simulink model "gm_sampleModel1787_sub"  (R2023a)
settings: Solver=VariableStepAuto  StartTime=0.0  StopTime=10.0  RelTol=1e-3
libraries: simulink x3, hdlsllib x1
settings Model: Creator=user1  LastModifiedBy=user1
settings OptimizationCC: BlockReduction=off  ConditionallyExecuteInputs=off
settings DebuggingCC: InheritedTsInSrcMsg=none

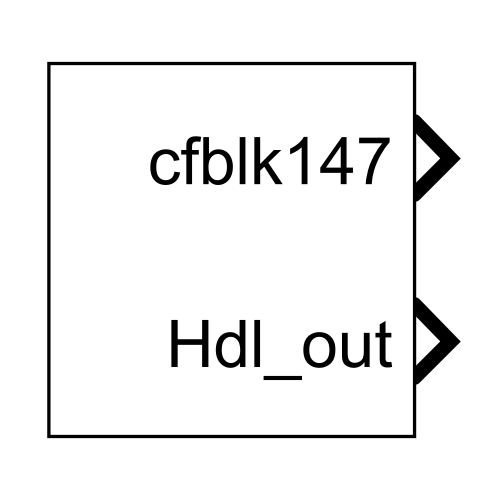
[thumbnail: Simulink's stored preview of the top-level diagram]
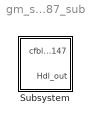
== system gm_sampleModel1787_sub ==
  Subsystem : Subsystem

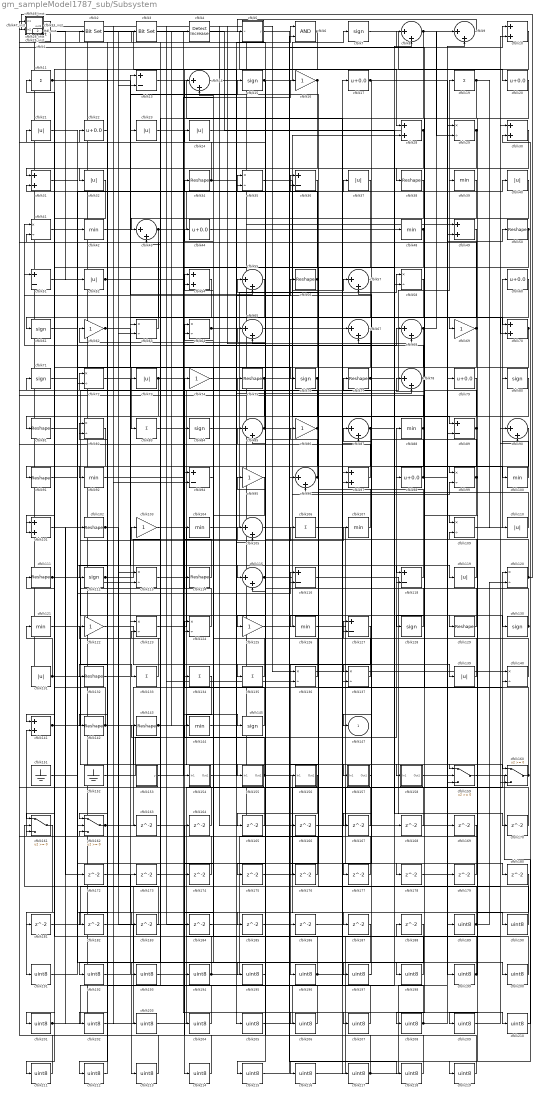
== system gm_sampleModel1787_sub/Subsystem ==
  cfblk1 : hdlsllib/Logic and Bit Operations/Bit Shift  mode=Shift Left Logical  N=0
  cfblk{10,28,30..31,49,54,70,97,101,141} (10 alike) : Sum  OutDataTypeStr=uint8
  cfblk{39,42,48,88,92,100,104,107,121,126,144} (11 alike) : MinMax  OutDataTypeStr=uint8
  cfblk{34,38,50,56,75,77,81,91,102,111,114,129,132,142..143} (15 alike) : Reshape
  cfblk{16,62,69,74,86,95,103,122,125} (9 alike) : Gain  OutDataTypeStr=uint8
  cfblk{8..9,14,43,55,57,65,67..68,78,85,87,90,96,105,115} (16 alike) : Sum  Inputs=|++  OutDataTypeStr=uint8
  cfblk{11,19,83,106,133..135} (7 alike) : Sum  Inputs=+  OutDataTypeStr=uint8
  cfblk108_inst : Subsystem
  cfblk{29,35,41,58,63..64,72,82,99,109,113,120,123..124,136..137,140} (17 alike) : Product  Inputs=*/  OutDataTypeStr=uint8  RndMeth=Zero  SaturateOnIntegerOverflow=on
  cfblk{21,23..24,32,37,40,52,73,110,119,131,139} (12 alike) : Abs  OutDataTypeStr=uint8  SaturateOnIntegerOverflow=off
  cfblk{7,15,61,71,76,80,84,112,128,130,145} (11 alike) : Signum
  cfblk{13,36,51,89,94,116,118,127} (8 alike) : Sum  Inputs=+-  OutDataTypeStr=uint8
  cfblk151 : Ground
  cfblk152 : Ground
  cfblk153 : Subsystem  mask(Counter Free-Running){NumBits=double(16), tsamp=double(-1)}
      mask prompts: NumBits "Simulink:masks:NumberOfBits_MP"; tsamp "Simulink:masks:SampleTime_MP"
      mask help: Simulink:masks:CounterFreeRunning_MD
  cfblk154 : Subsystem
  cfblk155 : Subsystem
  cfblk156 : Subsystem
  cfblk157 : Subsystem
  cfblk158 : Subsystem
  cfblk{159..162} (4 alike) : Switch  OutDataTypeStr=uint8  SaturateOnIntegerOverflow=off  InputSameDT=off
  cfblk{163..170,172..188} (25 alike) : Delay  SampleTime=1
  cfblk{17,20,22,44,60,79,98} (7 alike) : Bias  Bias=0.0  SaturateOnIntegerOverflow=off
  cfblk{189..219} (31 alike) : DataTypeConversion  OutDataTypeStr=uint8  SaturateOnIntegerOverflow=off  RndMeth=Floor
  cfblk18_inst : Subsystem
  cfblk2 : simulink/Logic and Bit Operations/Bit Set  iBit=0
      settings: LibrarySourceBlock=|
      | hdlsllib/Logic and Bit
      | Operations/Bit Set
  cfblk25_inst : Subsystem
  cfblk26_inst : Subsystem
  cfblk3 : simulink/Logic and Bit Operations/Bit Set  iBit=0
      settings: LibrarySourceBlock=|
      | hdlsllib/Logic and Bit
      | Operations/Bit Set
  cfblk33_inst : Subsystem
  cfblk4 : simulink/Logic and Bit Operations/Detect Increase  vinit=0.0  OutDataTypeStr=uint8
      settings: LibrarySourceBlock=|
      | hdlsllib/Logic and Bit
      | Operations/Detect
      | Increase
  cfblk46_inst : Subsystem
  cfblk47_inst : Subsystem
  cfblk5 : Subsystem  mask(Compare To Zero){relop=<=, OutDataTypeStr=uint8, ZeroCross=on}
      mask prompts: relop "Simulink:masks:Operator_MP"; OutDataTypeStr "Simulink:masks:OutputDataType_MP"; ZeroCross "Simulink:masks:EnableZerocrossingDetection_MP"
      mask help: Simulink:masks:CompareToZero_MD
      mask init:
      | OutDataTypeStr = 'uint8';
      | ZeroCross = 'on';
      | blkName = 'sampleModel1787_sub/Subsystem/cfblk5';
      | relop = '<=';
      | setValue = 'fixdt(0, 8)';
      mask TypeOptions relop: == | ~= | < | <= | >= | >
      mask TypeOptions OutDataTypeStr: Simulink:masks:uint8 | Simulink:masks:boolean
      mask Callback ZeroCross: sl('zeroCrossEnable', gcbh);
      mask Display: disp([relop,' 0'])
  cfblk6 : Logic  AllPortsSameDT=off  OutDataTypeStr=boolean
  cfblk147 : Outport  OutDataTypeStr=uint8  SampleTime=1  VectorParamsAs1DForOutWhenUnconnected=off
  Hdl_out : Outport  Port=2  OutDataTypeStr=uint8  SampleTime=1
  wires:
  cfblk1/1 -> cfblk52/1
  cfblk10/1 -> cfblk214/1
  cfblk100/1 -> cfblk60/1
  cfblk101/1 -> cfblk172/1
  cfblk102/1 -> cfblk13/2, cfblk173/1
  cfblk103/1 -> cfblk159/1
  cfblk104/1 -> cfblk58/1
  cfblk105/1 -> cfblk37/1
  cfblk106/1 -> cfblk139/1
  cfblk107/1 -> cfblk55/1
  cfblk108_inst/1(out1) -> cfblk68/2, cfblk169/1, cfblk168/1
  cfblk109/1 -> cfblk80/1
  cfblk11/1 -> cfblk55/2, cfblk23/1
  cfblk110/1 -> cfblk96/2
  cfblk111/1 -> cfblk75/1, cfblk129/1
  cfblk112/1 -> cfblk105/1, cfblk113/1
  cfblk113/1 -> cfblk107/1
  cfblk114/1 -> cfblk74/1
  cfblk115/1 -> cfblk57/1, cfblk99/2
  cfblk116/1 -> cfblk189/1
  cfblk118/1 -> cfblk13/1
  cfblk119/1 -> cfblk24/1
  cfblk120/1 -> cfblk47_inst/2(in2), cfblk62/1
  cfblk121/1 -> cfblk133/1
  cfblk122/1 -> cfblk199/1
  cfblk123/1 -> cfblk19/1
  cfblk124/1 -> cfblk104/1
  cfblk125/1 -> cfblk28/2
  cfblk126/1 -> cfblk180/1
  cfblk127/1 -> cfblk196/1
  cfblk128/1 -> cfblk88/1
  cfblk129/1 -> cfblk26_inst/1(in1)
  cfblk13/1 -> cfblk97/2
  cfblk130/1 -> cfblk77/1, cfblk72/1
  cfblk131/1 -> cfblk157/1(In1), cfblk121/1
  cfblk132/1 -> cfblk15/1
  cfblk133/1 -> cfblk22/1
  cfblk134/1 -> cfblk154/1(In1)
  cfblk135/1 -> cfblk14/2
  cfblk136/1 -> cfblk34/1
  cfblk137/1 -> cfblk14/1
  cfblk139/1 -> cfblk54/1
  cfblk14/1 -> cfblk69/1
  cfblk140/1 -> cfblk85/2
  cfblk141/1 -> cfblk114/1, cfblk106/1
  cfblk142/1 -> cfblk9/2, cfblk71/1, cfblk155/1(In1)
  cfblk143/1 -> cfblk145/1, cfblk4/1
  cfblk144/1 -> cfblk6/1
  cfblk145/1 -> cfblk124/1
  cfblk15/1 -> cfblk7/1, cfblk115/2
  cfblk151/1 -> cfblk42/1
  cfblk152/1 -> cfblk98/1
  cfblk153/1(y) -> cfblk16/1
  cfblk154/1(Out1) -> cfblk40/1
  cfblk155/1(Out1) -> cfblk187/1, cfblk144/1
  cfblk156/1(Out1) -> cfblk165/1
  cfblk157/1(Out1) -> cfblk87/1
  cfblk158/1(Out1) -> cfblk50/1
  cfblk159/1 -> cfblk216/1
  cfblk16/1 -> cfblk31/1, cfblk101/2
  cfblk160/1 -> cfblk78/1, cfblk67/2, cfblk86/1
  cfblk161/1 -> cfblk191/1
  cfblk162/1 -> cfblk118/2, cfblk63/2
  cfblk163/1 -> cfblk96/1
  cfblk164/1 -> cfblk46_inst/2(in2)
  cfblk165/1 -> cfblk25_inst/1(in1)
  cfblk166/1 -> cfblk120/1
  cfblk167/1 -> cfblk64/1
  cfblk168/1 -> cfblk85/1
  cfblk169/1 -> cfblk162/3
  cfblk17/1 -> cfblk79/1, cfblk57/2
  cfblk170/1 -> cfblk54/2
  cfblk172/1 -> cfblk190/1
  cfblk173/1 -> cfblk6/2
  cfblk174/1 -> cfblk63/1
  cfblk175/1 -> cfblk160/2
  cfblk176/1 -> cfblk141/2
  cfblk177/1 -> cfblk108_inst/2(in2)
  cfblk178/1 -> cfblk29/1
  cfblk179/1 -> cfblk161/3
  cfblk18_inst/1(out1) -> cfblk136/2
  cfblk180/1 -> cfblk209/1
  cfblk181/1 -> cfblk160/3
  cfblk182/1 -> cfblk198/1
  cfblk183/1 -> cfblk161/2
  cfblk184/1 -> cfblk1/1
  cfblk185/1 -> cfblk35/1
  cfblk186/1 -> cfblk140/2
  cfblk187/1 -> cfblk213/1
  cfblk188/1 -> cfblk192/1
  cfblk189/1 -> cfblk97/1, cfblk120/2
  cfblk19/1 -> cfblk38/1, cfblk110/1
  cfblk190/1 -> cfblk116/1
  cfblk191/1 -> cfblk116/2
  cfblk192/1 -> cfblk123/1
  cfblk193/1 -> cfblk188/1
  cfblk194/1 -> cfblk17/1, cfblk123/2
  cfblk195/1 -> cfblk95/1
  cfblk196/1 -> cfblk49/2, cfblk111/1
  cfblk197/1 -> cfblk127/1
  cfblk198/1 -> cfblk127/2
  cfblk199/1 -> cfblk109/2, cfblk134/1
  cfblk2/1 -> cfblk205/1
  cfblk20/1 -> cfblk109/1
  cfblk200/1 -> cfblk122/1
  cfblk201/1 -> cfblk87/2, cfblk102/1
  cfblk202/1 -> cfblk90/1
  cfblk203/1 -> cfblk90/2
  cfblk204/1 -> cfblk2/1
  cfblk205/1 -> cfblk48/1
  cfblk206/1 -> cfblk3/1
  cfblk207/1 -> cfblk103/1
  cfblk208/1 -> cfblk159/3, cfblk143/1
  cfblk209/1 -> cfblk30/1
  cfblk21/1 -> cfblk183/1
  cfblk210/1 -> cfblk30/2
  cfblk211/1 -> cfblk46_inst/1(in1)
  cfblk212/1 -> cfblk82/1
  cfblk213/1 -> cfblk82/2
  cfblk214/1 -> cfblk164/1
  cfblk215/1 -> cfblk10/1
  cfblk216/1 -> cfblk10/2
  cfblk217/1 -> cfblk18_inst/1(in1), cfblk179/1
  cfblk218/1 -> cfblk65/1
  cfblk219/1 -> cfblk65/2
  cfblk22/1 -> cfblk142/1
  cfblk23/1 -> cfblk200/1
  cfblk24/1 -> cfblk70/1
  cfblk25_inst/1(out1) -> cfblk131/1
  cfblk26_inst/1(out1) -> cfblk49/1
  cfblk28/1 -> cfblk32/1, Hdl_out/1
  cfblk29/1 -> cfblk61/1, cfblk219/1
  cfblk3/1 -> cfblk207/1
  cfblk30/1 -> cfblk208/1
  cfblk31/1 -> cfblk197/1
  cfblk32/1 -> cfblk141/1
  cfblk33_inst/1(out1) -> cfblk204/1, cfblk203/1, cfblk113/2
  cfblk34/1 -> cfblk33_inst/1(in1), cfblk105/2
  cfblk35/1 -> cfblk89/1
  cfblk36/1 -> cfblk181/1
  cfblk37/1 -> cfblk126/1
  cfblk38/1 -> cfblk193/1
  cfblk39/1 -> cfblk167/1
  cfblk4/1 -> cfblk28/1
  cfblk40/1 -> cfblk43/1
  cfblk41/1 -> cfblk39/1
  cfblk42/1 -> cfblk36/1
  cfblk43/1 -> cfblk36/2, cfblk112/1
  cfblk44/1 -> cfblk119/1
  cfblk46_inst/1(out1) -> cfblk163/1, cfblk140/1
  cfblk47_inst/1(out1) -> cfblk94/2, cfblk51/2, cfblk186/1
  cfblk48/1 -> cfblk176/1, cfblk137/1
  cfblk49/1 -> cfblk159/2
  cfblk5/1(y) -> cfblk158/1(In1)
  cfblk50/1 -> cfblk99/1, cfblk175/1
  cfblk51/1 -> cfblk185/1
  cfblk52/1 -> cfblk195/1, cfblk58/2
  cfblk54/1 -> cfblk64/2
  cfblk55/1 -> cfblk92/1
  cfblk56/1 -> cfblk21/1, cfblk184/1
  cfblk57/1 -> cfblk136/1
  cfblk58/1 -> cfblk166/1
  cfblk6/1 -> cfblk161/1, cfblk132/1
  cfblk60/1 -> cfblk91/1
  cfblk61/1 -> cfblk178/1
  cfblk62/1 -> cfblk76/1, cfblk70/2
  cfblk63/1 -> cfblk108_inst/1(in1)
  cfblk64/1 -> cfblk78/2, cfblk56/1, cfblk160/1
  cfblk65/1 -> cfblk217/1
  cfblk67/1 -> cfblk83/1
  cfblk68/1 -> cfblk94/1, cfblk9/1, cfblk72/2
  cfblk69/1 -> cfblk101/1, cfblk41/2
  cfblk7/1 -> cfblk20/1
  cfblk70/1 -> cfblk202/1, cfblk174/1, cfblk147/1
  cfblk71/1 -> cfblk73/1
  cfblk72/1 -> cfblk115/1
  cfblk73/1 -> cfblk162/1, cfblk135/1
  cfblk74/1 -> cfblk206/1
  cfblk75/1 -> cfblk67/1, cfblk218/1, cfblk212/1
  cfblk76/1 -> cfblk84/1, cfblk156/1(In1)
  cfblk77/1 -> cfblk8/2, cfblk100/1
  cfblk78/1 -> cfblk162/2, cfblk41/1
  cfblk79/1 -> cfblk215/1
  cfblk8/1 -> cfblk43/2, cfblk29/2
  cfblk80/1 -> cfblk81/1
  cfblk81/1 -> cfblk118/1
  cfblk82/1 -> cfblk211/1
  cfblk83/1 -> cfblk68/1
  cfblk84/1 -> cfblk210/1
  cfblk85/1 -> cfblk47_inst/1(in1), cfblk130/1
  cfblk86/1 -> cfblk182/1, cfblk11/1
  cfblk87/1 -> cfblk170/1, cfblk137/2
  cfblk88/1 -> cfblk33_inst/2(in2), cfblk177/1
  cfblk89/1 -> cfblk25_inst/2(in2), cfblk125/1
  cfblk9/1 -> cfblk5/1(u)
  cfblk90/1 -> cfblk201/1
  cfblk91/1 -> cfblk35/2
  cfblk92/1 -> cfblk124/2
  cfblk94/1 -> cfblk44/1
  cfblk95/1 -> cfblk194/1
  cfblk96/1 -> cfblk31/2, cfblk18_inst/2(in2)
  cfblk97/1 -> cfblk26_inst/2(in2)
  cfblk98/1 -> cfblk89/2, cfblk51/1
  cfblk99/1 -> cfblk8/1, cfblk128/1

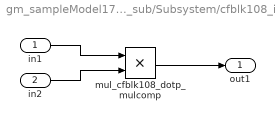
== system gm_sampleModel1787_sub/Subsystem/cfblk108_inst ==
  in1 : Inport  OutDataTypeStr=uint8  SampleTime=1
  in2 : Inport  Port=2  OutDataTypeStr=uint8  SampleTime=1
  mul_cfblk108_dotp_mulcomp : Product  Inputs=**  OutDataTypeStr=uint8  SampleTime=1
  out1 : Outport  OutDataTypeStr=uint8  SampleTime=1
  wires:
  in1/1 -> mul_cfblk108_dotp_mulcomp/1
  in2/1 -> mul_cfblk108_dotp_mulcomp/2
  mul_cfblk108_dotp_mulcomp/1 -> out1/1

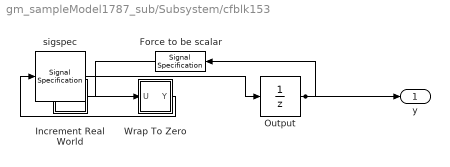
== system gm_sampleModel1787_sub/Subsystem/cfblk153 ==
  Force to be scalar : SignalSpecification  DisableCoverage=on  Dimensions=1
  Increment Real World : Subsystem  mask(Real World Value Increment){}
      mask help: Simulink:masks:RealWorldValueIncrement_MD
      mask Display: disp('V++')
  Output : UnitDelay  InitialCondition=0.0  SampleTime=tsamp  HasFrameUpgradeWarning=on
  Wrap To Zero : Subsystem  mask(Wrap To Zero){Threshold=double(65535)}
      mask prompts: Threshold "Simulink:masks:Threshold_MP"
      mask help: Simulink:masks:WrapToZero_MD
  sigspec : SignalSpecification  OutDataTypeStr=uint16  Dimensions=1
  y : Outport  SampleTime=1
  wires:
  Force to be scalar/1 -> Increment Real World/1(u)
  Increment Real World/1(y) -> Wrap To Zero/1(U)
  Output/1 -> Force to be scalar/1, y/1
  Wrap To Zero/1(Y) -> sigspec/1
  sigspec/1 -> Output/1

== system gm_sampleModel1787_sub/Subsystem/cfblk154 ==
  In1 : Inport  OutDataTypeStr=uint8  PortDimensions=1  SampleTime=1
  Out1 : Outport  SampleTime=1
  wires:
  In1/1 -> Out1/1

== system gm_sampleModel1787_sub/Subsystem/cfblk155 ==
  In1 : Inport  OutDataTypeStr=uint8  PortDimensions=1  SampleTime=1
  Out1 : Outport  SampleTime=1
  wires:
  In1/1 -> Out1/1

== system gm_sampleModel1787_sub/Subsystem/cfblk156 ==
  In1 : Inport  OutDataTypeStr=uint8  PortDimensions=1  SampleTime=1
  Out1 : Outport  SampleTime=1
  wires:
  In1/1 -> Out1/1

== system gm_sampleModel1787_sub/Subsystem/cfblk157 ==
  In1 : Inport  OutDataTypeStr=uint8  PortDimensions=1  SampleTime=1
  Out1 : Outport  SampleTime=1
  wires:
  In1/1 -> Out1/1

== system gm_sampleModel1787_sub/Subsystem/cfblk158 ==
  In1 : Inport  OutDataTypeStr=uint8  PortDimensions=1  SampleTime=1
  Out1 : Outport  SampleTime=1
  wires:
  In1/1 -> Out1/1

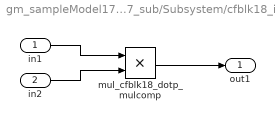
== system gm_sampleModel1787_sub/Subsystem/cfblk18_inst ==
  in1 : Inport  OutDataTypeStr=uint8  SampleTime=1
  in2 : Inport  Port=2  OutDataTypeStr=uint8  SampleTime=1
  mul_cfblk18_dotp_mulcomp : Product  Inputs=**  OutDataTypeStr=uint8  SampleTime=1
  out1 : Outport  OutDataTypeStr=uint8  SampleTime=1
  wires:
  in1/1 -> mul_cfblk18_dotp_mulcomp/1
  in2/1 -> mul_cfblk18_dotp_mulcomp/2
  mul_cfblk18_dotp_mulcomp/1 -> out1/1

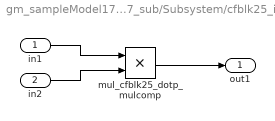
== system gm_sampleModel1787_sub/Subsystem/cfblk25_inst ==
  in1 : Inport  OutDataTypeStr=uint8  SampleTime=1
  in2 : Inport  Port=2  OutDataTypeStr=uint8  SampleTime=1
  mul_cfblk25_dotp_mulcomp : Product  Inputs=**  OutDataTypeStr=uint8  SampleTime=1
  out1 : Outport  OutDataTypeStr=uint8  SampleTime=1
  wires:
  in1/1 -> mul_cfblk25_dotp_mulcomp/1
  in2/1 -> mul_cfblk25_dotp_mulcomp/2
  mul_cfblk25_dotp_mulcomp/1 -> out1/1

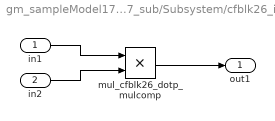
== system gm_sampleModel1787_sub/Subsystem/cfblk26_inst ==
  in1 : Inport  OutDataTypeStr=uint8  SampleTime=1
  in2 : Inport  Port=2  OutDataTypeStr=uint8  SampleTime=1
  mul_cfblk26_dotp_mulcomp : Product  Inputs=**  OutDataTypeStr=uint8  SampleTime=1
  out1 : Outport  OutDataTypeStr=uint8  SampleTime=1
  wires:
  in1/1 -> mul_cfblk26_dotp_mulcomp/1
  in2/1 -> mul_cfblk26_dotp_mulcomp/2
  mul_cfblk26_dotp_mulcomp/1 -> out1/1

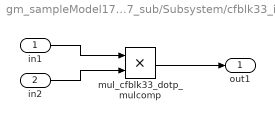
== system gm_sampleModel1787_sub/Subsystem/cfblk33_inst ==
  in1 : Inport  OutDataTypeStr=uint8  SampleTime=1
  in2 : Inport  Port=2  OutDataTypeStr=uint8  SampleTime=1
  mul_cfblk33_dotp_mulcomp : Product  Inputs=**  OutDataTypeStr=uint8  SampleTime=1
  out1 : Outport  OutDataTypeStr=uint8  SampleTime=1
  wires:
  in1/1 -> mul_cfblk33_dotp_mulcomp/1
  in2/1 -> mul_cfblk33_dotp_mulcomp/2
  mul_cfblk33_dotp_mulcomp/1 -> out1/1

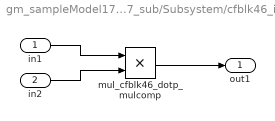
== system gm_sampleModel1787_sub/Subsystem/cfblk46_inst ==
  in1 : Inport  OutDataTypeStr=uint8  SampleTime=1
  in2 : Inport  Port=2  OutDataTypeStr=uint8  SampleTime=1
  mul_cfblk46_dotp_mulcomp : Product  Inputs=**  OutDataTypeStr=uint8  SampleTime=1
  out1 : Outport  OutDataTypeStr=uint8  SampleTime=1
  wires:
  in1/1 -> mul_cfblk46_dotp_mulcomp/1
  in2/1 -> mul_cfblk46_dotp_mulcomp/2
  mul_cfblk46_dotp_mulcomp/1 -> out1/1

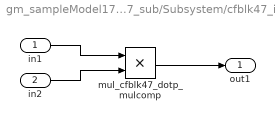
== system gm_sampleModel1787_sub/Subsystem/cfblk47_inst ==
  in1 : Inport  OutDataTypeStr=uint8  SampleTime=1
  in2 : Inport  Port=2  OutDataTypeStr=uint8  SampleTime=1
  mul_cfblk47_dotp_mulcomp : Product  Inputs=**  OutDataTypeStr=uint8  SampleTime=1
  out1 : Outport  OutDataTypeStr=uint8  SampleTime=1
  wires:
  in1/1 -> mul_cfblk47_dotp_mulcomp/1
  in2/1 -> mul_cfblk47_dotp_mulcomp/2
  mul_cfblk47_dotp_mulcomp/1 -> out1/1

== system gm_sampleModel1787_sub/Subsystem/cfblk5 ==
  u : Inport  OutDataTypeStr=uint8  SampleTime=1
  Compare : RelationalOperator  Operator=<=  OutDataTypeStr=fixdt(0, 8)
  Constant : Constant  DisableCoverage=on  Value=0  OutDataTypeStr=Inherit: Inherit via back propagation  SampleTime=-1  PreserveConstantTs=on
  y : Outport  SampleTime=1
  wires:
  u/1 -> Compare/1
  Compare/1 -> y/1
  Constant/1 -> Compare/2

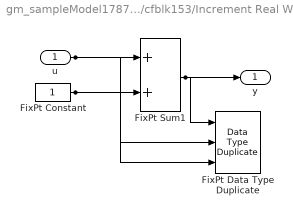
== system gm_sampleModel1787_sub/Subsystem/cfblk153/Increment Real World ==
  u : Inport  OutDataTypeStr=uint16  SampleTime=1
  FixPt Constant : Constant  DisableCoverage=on  OutDataTypeStr=Inherit: Inherit via back propagation  SampleTime=-1
  FixPt Data Type Duplicate : DataTypeDuplicate  DisableCoverage=on  NumInputPorts=3
  FixPt Sum1 : Sum  InputSameDT=on  OutDataTypeStr=Inherit: Inherit via back propagation  LockScale=on
  y : Outport  SampleTime=1
  wires:
  u/1 -> FixPt Sum1/1, FixPt Data Type Duplicate/2
  FixPt Constant/1 -> FixPt Sum1/2, FixPt Data Type Duplicate/3
  FixPt Sum1/1 -> FixPt Data Type Duplicate/1, y/1

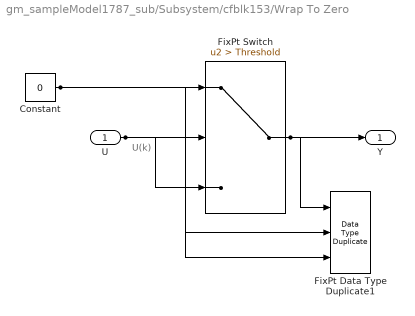
== system gm_sampleModel1787_sub/Subsystem/cfblk153/Wrap To Zero ==
  note: U(k)
  U : Inport  OutDataTypeStr=uint16  SampleTime=1
  Constant : Constant  DisableCoverage=on  Value=0  OutDataTypeStr=Inherit: Inherit via back propagation  SampleTime=-1
  FixPt Data Type Duplicate1 : DataTypeDuplicate  DisableCoverage=on  NumInputPorts=3
  FixPt Switch : Switch  Criteria=u2 > Threshold  Threshold=Threshold  OutDataTypeStr=Inherit: Inherit via back propagation  ZeroCross=off  SaturateOnIntegerOverflow=off  InputSameDT=off
  Y : Outport  SampleTime=1
  wires:
  U/1 -> FixPt Switch/3, FixPt Switch/2, FixPt Data Type Duplicate1/2
  Constant/1 -> FixPt Switch/1, FixPt Data Type Duplicate1/3
  FixPt Switch/1 -> FixPt Data Type Duplicate1/1, Y/1
